simulink model "NCO_Lab2"  (R2023a)
settings: Solver=VariableStepAuto  StartTime=0.0  StopTime=10.0  RelTol=1e-3
libraries: simulink x3
settings Model: Creator=v75u64  LastModifiedBy=mluser
settings DebuggingCC: UnconnectedInputMsg=warning  UnconnectedOutputMsg=warning  UnconnectedLineMsg=warning
settings ModelReferenceCC: EnableRefExpFcnMdlSchedulingChecks=on
settings RTWCC: DLArmComputeVersion=19.05

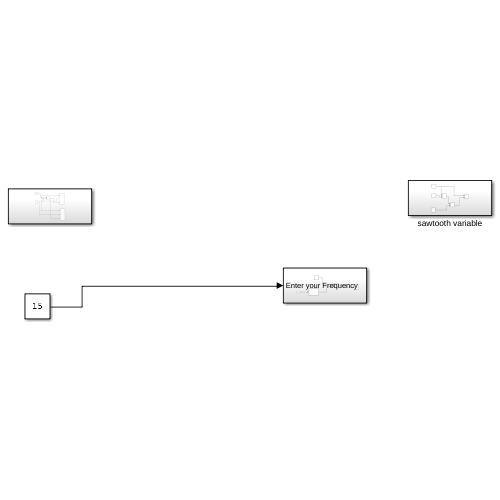
[thumbnail: Simulink's stored preview of the top-level diagram]
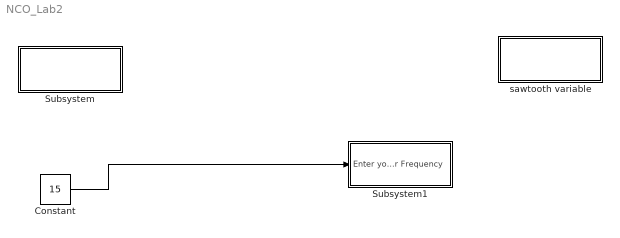
== system NCO_Lab2 ==
  Constant : Constant  Value=15
  Subsystem : Subsystem
  Subsystem1 : Subsystem
  sawtooth variable : Subsystem
  wires:
  Constant/1 -> Subsystem1/1(Enter your Frequency)

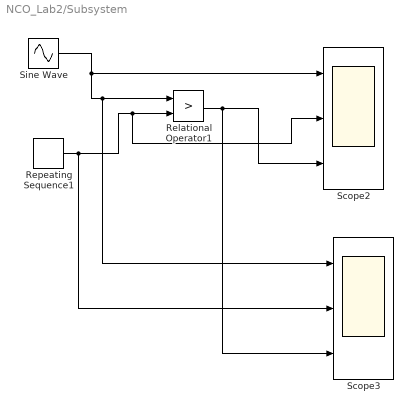
== system NCO_Lab2/Subsystem ==
  Relational Operator1 : RelationalOperator  Operator=>  OutDataTypeStr=boolean  RndMeth=Simplest  InputSameDT=off
  Repeating Sequence1 : simulink/Sources/Repeating Sequence  rep_seq_t=[0 0.5 1]  rep_seq_y=[0 2 0]
  Scope2 : Scope  NumInputPorts=3
  Scope3 : Scope  NumInputPorts=3
  Sine Wave : Sin  Frequency=0.5  SampleTime=0
  wires:
  Relational Operator1/1 -> Scope3/3, Scope2/3
  Sine Wave/1 -> Scope3/1, Relational Operator1/1, Scope2/1
  Repeating Sequence1/1 -> Scope3/2, Scope2/2, Relational Operator1/2

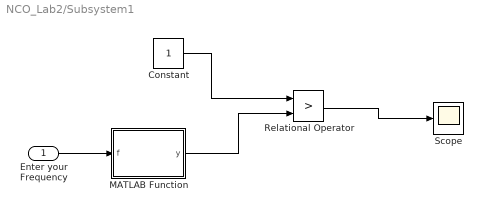
== system NCO_Lab2/Subsystem1 ==
  Enter your Frequency : Inport
  Constant : Constant
  MATLAB Function : MATLAB Function  TreatAsAtomicUnit=on
  Relational Operator : RelationalOperator  Operator=>  OutDataTypeStr=boolean  RndMeth=Simplest  InputSameDT=off
  Scope : Scope
  wires:
  Constant/1 -> Relational Operator/1
  MATLAB Function/1(y) -> Relational Operator/2
  Enter your Frequency/1 -> MATLAB Function/1(f)
  Relational Operator/1 -> Scope/1

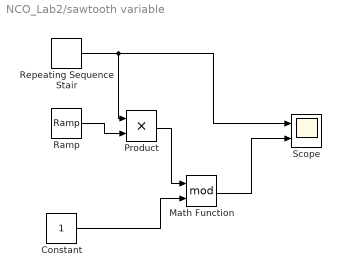
== system NCO_Lab2/sawtooth variable ==
  Constant : Constant  SampleTime=1
  Math Function : Math  Operator=mod
  Product : Product
  Ramp : simulink/Sources/Ramp  slope=1  start=0  InitialOutput=0
  Repeating Sequence Stair : simulink/Sources/Repeating Sequence Stair  OutValues=[1 2 3 4 5 6 5 4 3 2 1].'  tsamp=-1  OutMin=[]  OutMax=[]  OutDataTypeStr=double  OutputDataTypeScalingMode=double  OutDataType=fixdt(0,8)  ConRadixGroup=Best Precision: Vector-wise  OutScaling=2^-12
  Scope : Scope  NumInputPorts=2
  wires:
  Constant/1 -> Math Function/2
  Math Function/1 -> Scope/2
  Repeating Sequence Stair/1 -> Product/1, Scope/1
  Ramp/1 -> Product/2
  Product/1 -> Math Function/1

== matlab function NCO_Lab2/Subsystem1/MATLAB Function ==
  data: f input; y output
function y = variable_freq_sawtooth(f)
% Generate a variable frequency sawtooth waveform
% Inputs: f - the frequency of the sawtooth waveform (in Hz)
% Output: y - the generated waveform

% Define time vector
t = linspace(0, 1, 1000); % 1 second time interval, 1000 data points

% Generate sawtooth waveform
y = sawtooth(2*pi*f*t);

% Plot waveform (optional)
plot(t, y);
xlabel('Time (s)');
ylabel('Amplitude');
title(['Sawtooth Waveform with Frequency = ', ' Hz']);
grid on;

end
